simulink model "MVB1TestFlow"  (R2013b)
settings: Solver=ode45  StartTime=0.0  StopTime=6e-5  RelTol=1e-3
libraries: simulink x4
(part 1 of 2)
settings Model: Creator=qiji  LastModifiedBy=qiji
settings DataIOCC: SignalLoggingSaveFormat=ModelDataLogs
settings DebuggingCC: UnderspecifiedInitializationDetection=Simplified  MultiTaskDSMMsg=warning  MultiTaskCondExecSysMsg=none  SFUnusedDataAndEventsDiag=none
settings RTWCC: IncludeERTFirstTime=on
settings GRTTargetCC: CodeReplacementLibrary=None  CPPClassGenCompliant=on

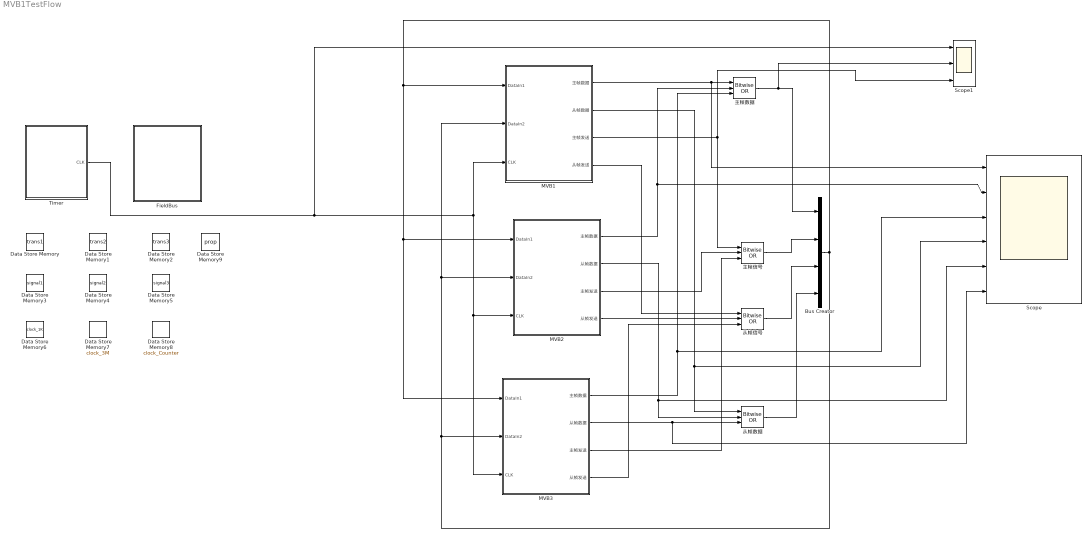
== system MVB1TestFlow ==
  Bus Creator : BusCreator
  Data Store Memory : DataStoreMemory  DataStoreName=trans1  ReadBeforeWriteMsg=warning  WriteAfterWriteMsg=warning  WriteAfterReadMsg=warning  OutDataTypeStr=boolean
  Data Store Memory1 : DataStoreMemory  DataStoreName=trans2  ReadBeforeWriteMsg=warning  WriteAfterWriteMsg=warning  WriteAfterReadMsg=warning  OutDataTypeStr=boolean
  Data Store Memory2 : DataStoreMemory  DataStoreName=trans3  ReadBeforeWriteMsg=warning  WriteAfterWriteMsg=warning  WriteAfterReadMsg=warning  OutDataTypeStr=boolean
  Data Store Memory3 : DataStoreMemory  DataStoreName=signal1  ReadBeforeWriteMsg=warning  WriteAfterWriteMsg=warning  WriteAfterReadMsg=warning  OutDataTypeStr=boolean
  Data Store Memory4 : DataStoreMemory  DataStoreName=signal2  ReadBeforeWriteMsg=warning  WriteAfterWriteMsg=warning  WriteAfterReadMsg=warning  OutDataTypeStr=boolean
  Data Store Memory5 : DataStoreMemory  DataStoreName=signal3  ReadBeforeWriteMsg=warning  WriteAfterWriteMsg=warning  WriteAfterReadMsg=warning  OutDataTypeStr=boolean
  Data Store Memory6 : DataStoreMemory  DataStoreName=clock_1K  ReadBeforeWriteMsg=warning  WriteAfterWriteMsg=warning  WriteAfterReadMsg=warning  OutDataTypeStr=boolean
  Data Store Memory7 : DataStoreMemory  DataStoreName=clock_3M  ReadBeforeWriteMsg=warning  WriteAfterWriteMsg=warning  WriteAfterReadMsg=warning  OutDataTypeStr=boolean
  Data Store Memory8 : DataStoreMemory  DataStoreName=clock_Counter  ReadBeforeWriteMsg=warning  WriteAfterWriteMsg=warning  WriteAfterReadMsg=warning  OutDataTypeStr=uint32
  Data Store Memory9 : DataStoreMemory  DataStoreName=prop  ReadBeforeWriteMsg=warning  WriteAfterWriteMsg=warning  WriteAfterReadMsg=warning  InitialValue=10  OutDataTypeStr=double
  FieldBus : Subsystem
  MVB1 : Subsystem
  MVB2 : Subsystem
  MVB3 : Subsystem
  Scope : Scope  NumInputPorts=6
      settings: YMin=0~0~0~0~0~0  YMax=3e+09~3e+09~3e+09~3e+09~3000000000~3e+09
  Scope1 : Scope  NumInputPorts=3
      settings: YMin=-5~-5~-5  YMax=5~5~5
  Timer : Subsystem
  主帧信号 : simulink/Logic and Bit Operations/Bitwise Operator  logicop=OR  UseBitMask=off  NumInputPorts=3  BitMask=bin2dec('11011001')  BitMaskRealWorld=Stored Integer
  主帧数据 : simulink/Logic and Bit Operations/Bitwise Operator  logicop=OR  UseBitMask=off  NumInputPorts=3  BitMask=bin2dec('11011001')  BitMaskRealWorld=Stored Integer
  从帧信号 : simulink/Logic and Bit Operations/Bitwise Operator  logicop=OR  UseBitMask=off  NumInputPorts=3  BitMask=bin2dec('11011001')  BitMaskRealWorld=Stored Integer
  从帧数据 : simulink/Logic and Bit Operations/Bitwise Operator  logicop=OR  UseBitMask=off  NumInputPorts=3  BitMask=bin2dec('11011001')  BitMaskRealWorld=Stored Integer
  wires:
  MVB1/1(主帧数据) -> Scope/1, 主帧数据/1
  MVB2/1(主帧数据) -> Scope/2, 主帧数据/2
  MVB3/1(主帧数据) -> Scope/3, 主帧数据/3
  MVB1/2(从帧数据) -> Scope/4, 从帧数据/1
  MVB2/2(从帧数据) -> Scope/5, 从帧数据/2
  MVB3/2(从帧数据) -> Scope/6, 从帧数据/3
  MVB1/3(主帧发送) -> 主帧信号/1, Scope1/3
  MVB2/3(主帧发送) -> 主帧信号/2
  MVB3/3(主帧发送) -> 主帧信号/3
  MVB1/4(从帧发送) -> 从帧信号/1
  MVB2/4(从帧发送) -> 从帧信号/2
  MVB3/4(从帧发送) -> 从帧信号/3
  主帧数据/1 -> Scope1/2, Bus Creator/1
  主帧信号/1 -> Bus Creator/2
  从帧信号/1 -> Bus Creator/3
  从帧数据/1 -> Bus Creator/4
  Bus Creator/1 -> MVB3/1(DataIn1), MVB2/1(DataIn1), MVB1/1(DataIn1), MVB3/2(DataIn2), MVB1/2(DataIn2), MVB2/2(DataIn2)
  Timer/1(CLK) -> Scope1/1, MVB1/3(CLK), MVB3/3(CLK), MVB2/3(CLK)

== system MVB1TestFlow/FieldBus ==
  FIELDBUS : Stateflow chart  TreatAsAtomicUnit=on

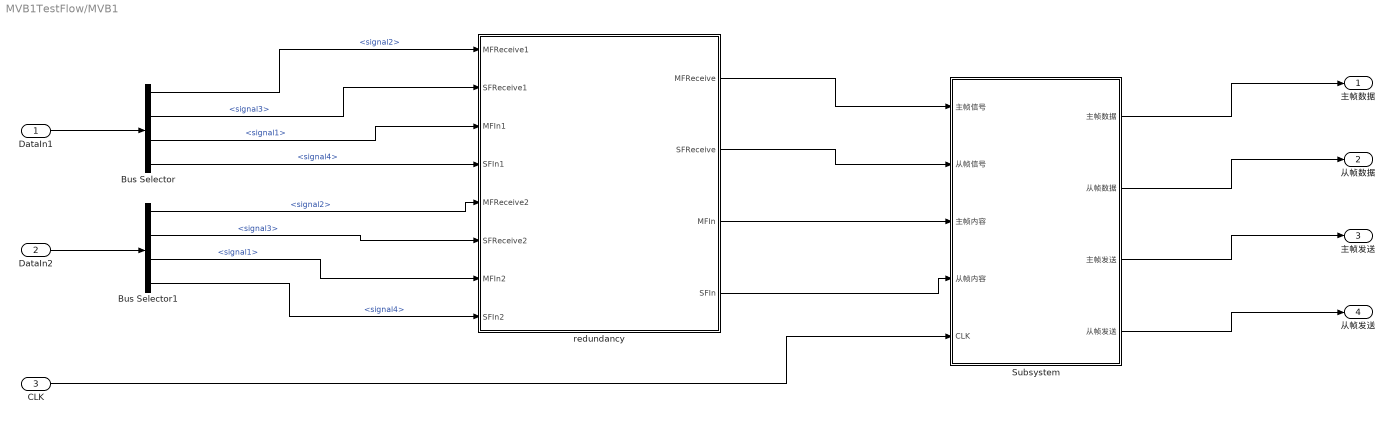
== system MVB1TestFlow/MVB1 ==
  DataIn1 : Inport  PortDimensions=4
  DataIn2 : Inport  Port=2  PortDimensions=4
  CLK : Inport  Port=3
  Bus Selector : BusSelector  OutputSignals=signal2,signal3,signal1,signal4
  Bus Selector1 : BusSelector  OutputSignals=signal2,signal3,signal1,signal4
  Subsystem : Subsystem
  redundancy : Stateflow chart  TreatAsAtomicUnit=on
  主帧数据 : Outport
  从帧数据 : Outport  Port=2
  主帧发送 : Outport  Port=3
  从帧发送 : Outport  Port=4
  wires:
  Subsystem/1(主帧数据) -> 主帧数据/1
  Subsystem/2(从帧数据) -> 从帧数据/1
  Subsystem/3(主帧发送) -> 主帧发送/1
  Subsystem/4(从帧发送) -> 从帧发送/1
  DataIn1/1 -> Bus Selector/1
  Bus Selector/3 -> redundancy/3(MFIn1)  "<signal1>"
  Bus Selector/1 -> redundancy/1(MFReceive1)  "<signal2>"
  Bus Selector/2 -> redundancy/2(SFReceive1)  "<signal3>"
  Bus Selector/4 -> redundancy/4(SFIn1)  "<signal4>"
  DataIn2/1 -> Bus Selector1/1
  redundancy/1(MFReceive) -> Subsystem/1(主帧信号)
  redundancy/2(SFReceive) -> Subsystem/2(从帧信号)
  redundancy/3(MFIn) -> Subsystem/3(主帧内容)
  redundancy/4(SFIn) -> Subsystem/4(从帧内容)
  Bus Selector1/1 -> redundancy/5(MFReceive2)  "<signal2>"
  Bus Selector1/2 -> redundancy/6(SFReceive2)  "<signal3>"
  Bus Selector1/3 -> redundancy/7(MFIn2)  "<signal1>"
  Bus Selector1/4 -> redundancy/8(SFIn2)  "<signal4>"
  CLK/1 -> Subsystem/5(CLK)

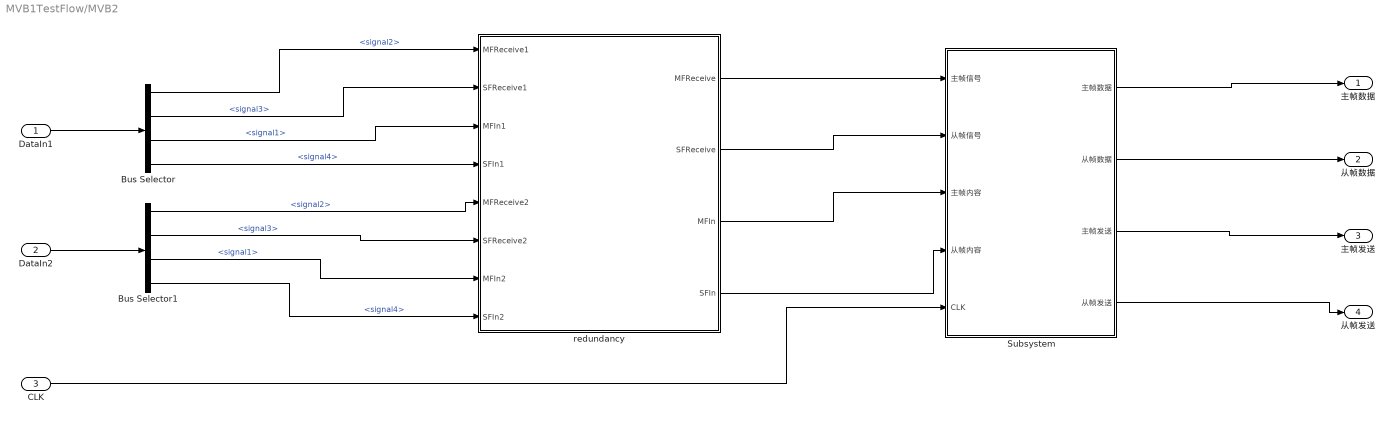
== system MVB1TestFlow/MVB2 ==
  DataIn1 : Inport  PortDimensions=4
  DataIn2 : Inport  Port=2  PortDimensions=4
  CLK : Inport  Port=3
  Bus Selector : BusSelector  OutputSignals=signal2,signal3,signal1,signal4
  Bus Selector1 : BusSelector  OutputSignals=signal2,signal3,signal1,signal4
  Subsystem : Subsystem
  redundancy : Stateflow chart  TreatAsAtomicUnit=on
  主帧数据 : Outport
  从帧数据 : Outport  Port=2
  主帧发送 : Outport  Port=3
  从帧发送 : Outport  Port=4
  wires:
  Subsystem/1(主帧数据) -> 主帧数据/1
  Subsystem/2(从帧数据) -> 从帧数据/1
  Subsystem/3(主帧发送) -> 主帧发送/1
  Subsystem/4(从帧发送) -> 从帧发送/1
  DataIn1/1 -> Bus Selector/1
  Bus Selector/3 -> redundancy/3(MFIn1)  "<signal1>"
  Bus Selector/1 -> redundancy/1(MFReceive1)  "<signal2>"
  Bus Selector/2 -> redundancy/2(SFReceive1)  "<signal3>"
  Bus Selector/4 -> redundancy/4(SFIn1)  "<signal4>"
  DataIn2/1 -> Bus Selector1/1
  redundancy/1(MFReceive) -> Subsystem/1(主帧信号)
  redundancy/2(SFReceive) -> Subsystem/2(从帧信号)
  redundancy/3(MFIn) -> Subsystem/3(主帧内容)
  redundancy/4(SFIn) -> Subsystem/4(从帧内容)
  Bus Selector1/1 -> redundancy/5(MFReceive2)  "<signal2>"
  Bus Selector1/2 -> redundancy/6(SFReceive2)  "<signal3>"
  Bus Selector1/3 -> redundancy/7(MFIn2)  "<signal1>"
  Bus Selector1/4 -> redundancy/8(SFIn2)  "<signal4>"
  CLK/1 -> Subsystem/5(CLK)

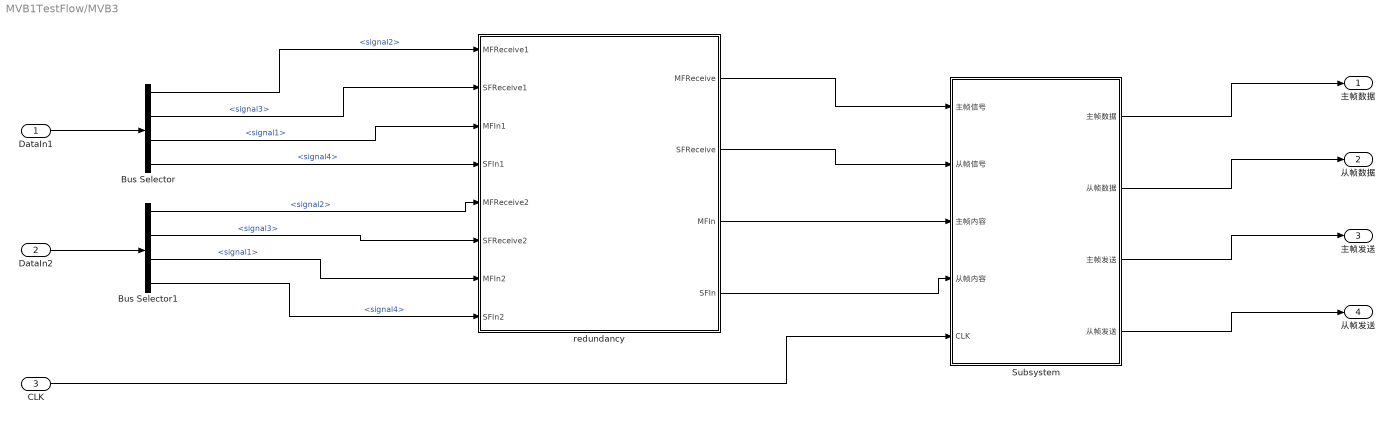
== system MVB1TestFlow/MVB3 ==
  DataIn1 : Inport  PortDimensions=4
  DataIn2 : Inport  Port=2  PortDimensions=4
  CLK : Inport  Port=3
  Bus Selector : BusSelector  OutputSignals=signal2,signal3,signal1,signal4
  Bus Selector1 : BusSelector  OutputSignals=signal2,signal3,signal1,signal4
  Subsystem : Subsystem
  redundancy : Stateflow chart  TreatAsAtomicUnit=on
  主帧数据 : Outport
  从帧数据 : Outport  Port=2
  主帧发送 : Outport  Port=3
  从帧发送 : Outport  Port=4
  wires:
  Subsystem/1(主帧数据) -> 主帧数据/1
  Subsystem/2(从帧数据) -> 从帧数据/1
  Subsystem/3(主帧发送) -> 主帧发送/1
  Subsystem/4(从帧发送) -> 从帧发送/1
  DataIn1/1 -> Bus Selector/1
  Bus Selector/3 -> redundancy/3(MFIn1)  "<signal1>"
  Bus Selector/1 -> redundancy/1(MFReceive1)  "<signal2>"
  Bus Selector/2 -> redundancy/2(SFReceive1)  "<signal3>"
  Bus Selector/4 -> redundancy/4(SFIn1)  "<signal4>"
  DataIn2/1 -> Bus Selector1/1
  redundancy/1(MFReceive) -> Subsystem/1(主帧信号)
  redundancy/2(SFReceive) -> Subsystem/2(从帧信号)
  redundancy/3(MFIn) -> Subsystem/3(主帧内容)
  redundancy/4(SFIn) -> Subsystem/4(从帧内容)
  Bus Selector1/1 -> redundancy/5(MFReceive2)  "<signal2>"
  Bus Selector1/2 -> redundancy/6(SFReceive2)  "<signal3>"
  Bus Selector1/3 -> redundancy/7(MFIn2)  "<signal1>"
  Bus Selector1/4 -> redundancy/8(SFIn2)  "<signal4>"
  CLK/1 -> Subsystem/5(CLK)

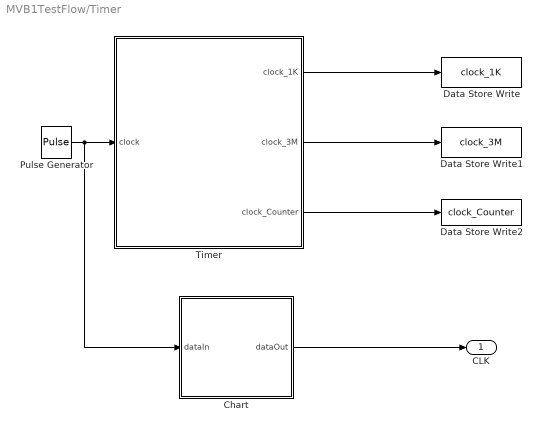
== system MVB1TestFlow/Timer ==
  Chart : Stateflow chart  TreatAsAtomicUnit=on
  Data Store Write : DataStoreWrite  DataStoreName=clock_1K
  Data Store Write1 : DataStoreWrite  DataStoreName=clock_3M
  Data Store Write2 : DataStoreWrite  DataStoreName=clock_Counter
  Pulse Generator : DiscretePulseGenerator  PulseType=Time based  Period=4.1666666667e-8  PulseWidth=50
  Timer : Stateflow chart  TreatAsAtomicUnit=on
  CLK : Outport  OutDataTypeStr=double
  wires:
  Timer/3(clock_Counter) -> Data Store Write2/1
  Timer/2(clock_3M) -> Data Store Write1/1
  Timer/1(clock_1K) -> Data Store Write/1
  Pulse Generator/1 -> Chart/1(dataIn), Timer/1(clock)
  Chart/1(dataOut) -> CLK/1

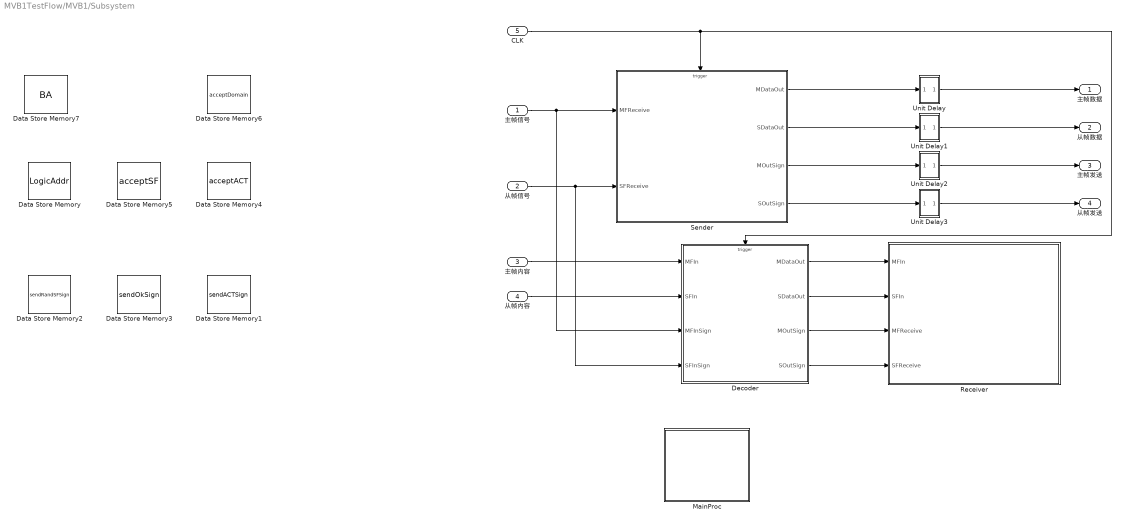
== system MVB1TestFlow/MVB1/Subsystem ==
  主帧信号 : Inport
  从帧信号 : Inport  Port=2
  主帧内容 : Inport  Port=3
  从帧内容 : Inport  Port=4
  CLK : Inport  Port=5
  Data Store Memory : DataStoreMemory  DataStoreName=LogicAddr  ReadBeforeWriteMsg=warning  WriteAfterWriteMsg=warning  WriteAfterReadMsg=warning  InitialValue=1  OutDataTypeStr=uint32
  Data Store Memory1 : DataStoreMemory  DataStoreName=sendACTSign  ReadBeforeWriteMsg=warning  WriteAfterWriteMsg=warning  WriteAfterReadMsg=warning  OutDataTypeStr=boolean
  Data Store Memory2 : DataStoreMemory  DataStoreName=sendRandSFSign  ReadBeforeWriteMsg=warning  WriteAfterWriteMsg=warning  WriteAfterReadMsg=warning  OutDataTypeStr=boolean
  Data Store Memory3 : DataStoreMemory  DataStoreName=sendOkSign  ReadBeforeWriteMsg=warning  WriteAfterWriteMsg=warning  WriteAfterReadMsg=warning  OutDataTypeStr=boolean
  Data Store Memory4 : DataStoreMemory  DataStoreName=acceptACT  ReadBeforeWriteMsg=warning  WriteAfterWriteMsg=warning  WriteAfterReadMsg=warning  InitialValue=false  OutDataTypeStr=boolean
  Data Store Memory5 : DataStoreMemory  DataStoreName=acceptSF  ReadBeforeWriteMsg=warning  WriteAfterWriteMsg=warning  WriteAfterReadMsg=warning  InitialValue=false  OutDataTypeStr=boolean
  Data Store Memory6 : DataStoreMemory  DataStoreName=acceptDomain  ReadBeforeWriteMsg=warning  WriteAfterWriteMsg=warning  WriteAfterReadMsg=warning  InitialValue=false  OutDataTypeStr=boolean
  Data Store Memory7 : DataStoreMemory  DataStoreName=BA  ReadBeforeWriteMsg=warning  WriteAfterWriteMsg=warning  WriteAfterReadMsg=warning  InitialValue=true  OutDataTypeStr=boolean
  Decoder : Stateflow chart  TreatAsAtomicUnit=on
  MainProc : Stateflow chart  TreatAsAtomicUnit=on
  Receiver : Stateflow chart  TreatAsAtomicUnit=on
  Sender : Stateflow chart  TreatAsAtomicUnit=on
  Unit Delay : Subsystem
  Unit Delay1 : Subsystem
  Unit Delay2 : Subsystem
  Unit Delay3 : Subsystem
  主帧数据 : Outport
  从帧数据 : Outport  Port=2
  主帧发送 : Outport  Port=3
  从帧发送 : Outport  Port=4
  wires:
  主帧信号/1 -> Decoder/3(MFInSign), Sender/1(MFReceive)
  Sender/3(MOutSign) -> Unit Delay2/1(In1)
  Sender/2(SDataOut) -> Unit Delay1/1(In1)
  Unit Delay3/1(Out) -> 从帧发送/1
  从帧信号/1 -> Decoder/4(SFInSign), Sender/2(SFReceive)
  Unit Delay1/1(Out) -> 从帧数据/1
  Sender/4(SOutSign) -> Unit Delay3/1(In1)
  从帧内容/1 -> Decoder/2(SFIn)
  Sender/1(MDataOut) -> Unit Delay/1(In1)
  Unit Delay2/1(Out) -> 主帧发送/1
  主帧内容/1 -> Decoder/1(MFIn)
  CLK/1 -> Decoder/Trigger, Sender/Trigger
  Decoder/1(MDataOut) -> Receiver/1(MFIn)
  Decoder/2(SDataOut) -> Receiver/2(SFIn)
  Decoder/3(MOutSign) -> Receiver/3(MFReceive)
  Decoder/4(SOutSign) -> Receiver/4(SFReceive)
  Unit Delay/1(Out) -> 主帧数据/1

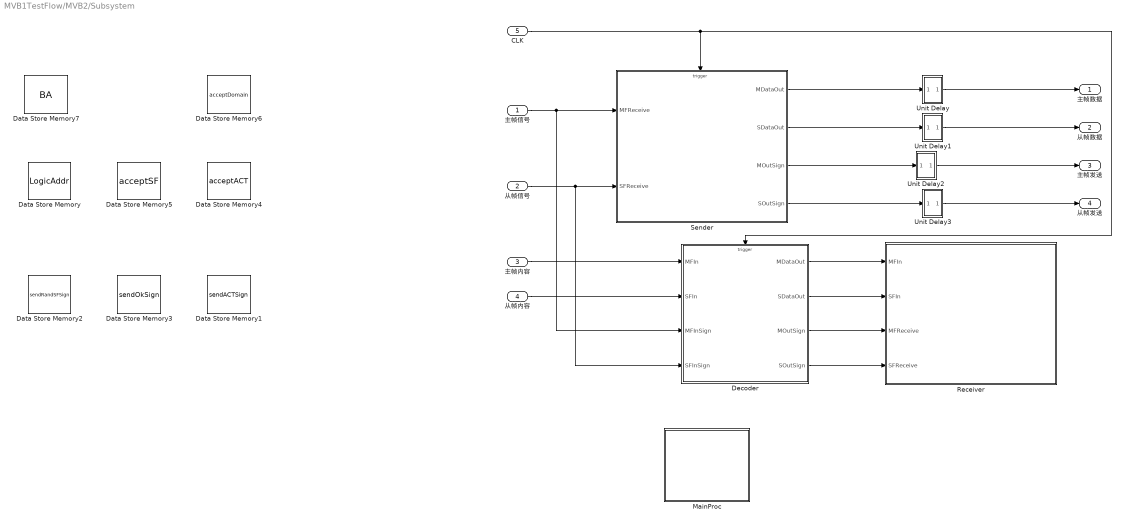
== system MVB1TestFlow/MVB2/Subsystem ==
  主帧信号 : Inport
  从帧信号 : Inport  Port=2
  主帧内容 : Inport  Port=3
  从帧内容 : Inport  Port=4
  CLK : Inport  Port=5
  Data Store Memory : DataStoreMemory  DataStoreName=LogicAddr  ReadBeforeWriteMsg=warning  WriteAfterWriteMsg=warning  WriteAfterReadMsg=warning  InitialValue=2  OutDataTypeStr=uint32
  Data Store Memory1 : DataStoreMemory  DataStoreName=sendACTSign  ReadBeforeWriteMsg=warning  WriteAfterWriteMsg=warning  WriteAfterReadMsg=warning  OutDataTypeStr=boolean
  Data Store Memory2 : DataStoreMemory  DataStoreName=sendRandSFSign  ReadBeforeWriteMsg=warning  WriteAfterWriteMsg=warning  WriteAfterReadMsg=warning  OutDataTypeStr=boolean
  Data Store Memory3 : DataStoreMemory  DataStoreName=sendOkSign  ReadBeforeWriteMsg=warning  WriteAfterWriteMsg=warning  WriteAfterReadMsg=warning  OutDataTypeStr=boolean
  Data Store Memory4 : DataStoreMemory  DataStoreName=acceptACT  ReadBeforeWriteMsg=warning  WriteAfterWriteMsg=warning  WriteAfterReadMsg=warning  InitialValue=false  OutDataTypeStr=boolean
  Data Store Memory5 : DataStoreMemory  DataStoreName=acceptSF  ReadBeforeWriteMsg=warning  WriteAfterWriteMsg=warning  WriteAfterReadMsg=warning  InitialValue=false  OutDataTypeStr=boolean
  Data Store Memory6 : DataStoreMemory  DataStoreName=acceptDomain  ReadBeforeWriteMsg=warning  WriteAfterWriteMsg=warning  WriteAfterReadMsg=warning  InitialValue=false  OutDataTypeStr=boolean
  Data Store Memory7 : DataStoreMemory  DataStoreName=BA  ReadBeforeWriteMsg=warning  WriteAfterWriteMsg=warning  WriteAfterReadMsg=warning  InitialValue=true  OutDataTypeStr=boolean
  Decoder : Stateflow chart  TreatAsAtomicUnit=on
  MainProc : Stateflow chart  TreatAsAtomicUnit=on
  Receiver : Stateflow chart  TreatAsAtomicUnit=on
  Sender : Stateflow chart  TreatAsAtomicUnit=on
  Unit Delay : Subsystem
  Unit Delay1 : Subsystem
  Unit Delay2 : Subsystem
  Unit Delay3 : Subsystem
  主帧数据 : Outport
  从帧数据 : Outport  Port=2
  主帧发送 : Outport  Port=3
  从帧发送 : Outport  Port=4
  wires:
  主帧信号/1 -> Decoder/3(MFInSign), Sender/1(MFReceive)
  Sender/3(MOutSign) -> Unit Delay2/1(In1)
  Sender/2(SDataOut) -> Unit Delay1/1(In1)
  Unit Delay3/1(Out) -> 从帧发送/1
  从帧信号/1 -> Decoder/4(SFInSign), Sender/2(SFReceive)
  Unit Delay1/1(Out) -> 从帧数据/1
  Sender/4(SOutSign) -> Unit Delay3/1(In1)
  从帧内容/1 -> Decoder/2(SFIn)
  Sender/1(MDataOut) -> Unit Delay/1(In1)
  Unit Delay/1(Out) -> 主帧数据/1
  Unit Delay2/1(Out) -> 主帧发送/1
  主帧内容/1 -> Decoder/1(MFIn)
  CLK/1 -> Decoder/Trigger, Sender/Trigger
  Decoder/1(MDataOut) -> Receiver/1(MFIn)
  Decoder/2(SDataOut) -> Receiver/2(SFIn)
  Decoder/3(MOutSign) -> Receiver/3(MFReceive)
  Decoder/4(SOutSign) -> Receiver/4(SFReceive)

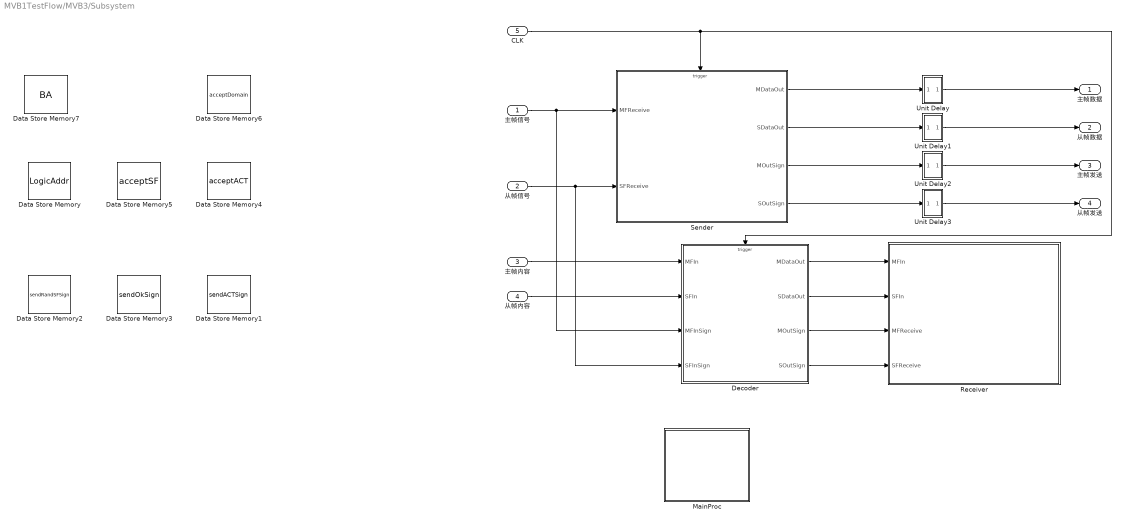
== system MVB1TestFlow/MVB3/Subsystem ==
  主帧信号 : Inport
  从帧信号 : Inport  Port=2
  主帧内容 : Inport  Port=3
  从帧内容 : Inport  Port=4
  CLK : Inport  Port=5
  Data Store Memory : DataStoreMemory  DataStoreName=LogicAddr  ReadBeforeWriteMsg=warning  WriteAfterWriteMsg=warning  WriteAfterReadMsg=warning  InitialValue=3  OutDataTypeStr=uint32
  Data Store Memory1 : DataStoreMemory  DataStoreName=sendACTSign  ReadBeforeWriteMsg=warning  WriteAfterWriteMsg=warning  WriteAfterReadMsg=warning  OutDataTypeStr=boolean
  Data Store Memory2 : DataStoreMemory  DataStoreName=sendRandSFSign  ReadBeforeWriteMsg=warning  WriteAfterWriteMsg=warning  WriteAfterReadMsg=warning  OutDataTypeStr=boolean
  Data Store Memory3 : DataStoreMemory  DataStoreName=sendOkSign  ReadBeforeWriteMsg=warning  WriteAfterWriteMsg=warning  WriteAfterReadMsg=warning  OutDataTypeStr=boolean
  Data Store Memory4 : DataStoreMemory  DataStoreName=acceptACT  ReadBeforeWriteMsg=warning  WriteAfterWriteMsg=warning  WriteAfterReadMsg=warning  InitialValue=false  OutDataTypeStr=boolean
  Data Store Memory5 : DataStoreMemory  DataStoreName=acceptSF  ReadBeforeWriteMsg=warning  WriteAfterWriteMsg=warning  WriteAfterReadMsg=warning  InitialValue=false  OutDataTypeStr=boolean
  Data Store Memory6 : DataStoreMemory  DataStoreName=acceptDomain  ReadBeforeWriteMsg=warning  WriteAfterWriteMsg=warning  WriteAfterReadMsg=warning  InitialValue=false  OutDataTypeStr=boolean
  Data Store Memory7 : DataStoreMemory  DataStoreName=BA  ReadBeforeWriteMsg=warning  WriteAfterWriteMsg=warning  WriteAfterReadMsg=warning  InitialValue=true  OutDataTypeStr=boolean
  Decoder : Stateflow chart  TreatAsAtomicUnit=on
  MainProc : Stateflow chart  TreatAsAtomicUnit=on
  Receiver : Stateflow chart  TreatAsAtomicUnit=on
  Sender : Stateflow chart  TreatAsAtomicUnit=on
  Unit Delay : Subsystem
  Unit Delay1 : Subsystem
  Unit Delay2 : Subsystem
  Unit Delay3 : Subsystem
  主帧数据 : Outport
  从帧数据 : Outport  Port=2
  主帧发送 : Outport  Port=3
  从帧发送 : Outport  Port=4
  wires:
  主帧信号/1 -> Decoder/3(MFInSign), Sender/1(MFReceive)
  Sender/3(MOutSign) -> Unit Delay2/1(In1)
  Sender/2(SDataOut) -> Unit Delay1/1(In1)
  Unit Delay3/1(Out) -> 从帧发送/1
  从帧信号/1 -> Decoder/4(SFInSign), Sender/2(SFReceive)
  Unit Delay1/1(Out) -> 从帧数据/1
  Sender/4(SOutSign) -> Unit Delay3/1(In1)
  从帧内容/1 -> Decoder/2(SFIn)
  Sender/1(MDataOut) -> Unit Delay/1(In1)
  Unit Delay/1(Out) -> 主帧数据/1
  Unit Delay2/1(Out) -> 主帧发送/1
  主帧内容/1 -> Decoder/1(MFIn)
  CLK/1 -> Decoder/Trigger, Sender/Trigger
  Decoder/1(MDataOut) -> Receiver/1(MFIn)
  Decoder/2(SDataOut) -> Receiver/2(SFIn)
  Decoder/3(MOutSign) -> Receiver/3(MFReceive)
  Decoder/4(SOutSign) -> Receiver/4(SFReceive)

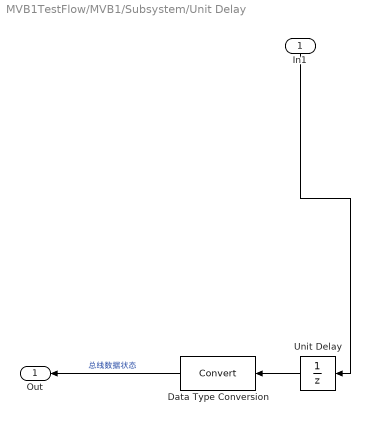
== system MVB1TestFlow/MVB1/Subsystem/Unit Delay ==
  In1 : Inport
  Data Type Conversion : DataTypeConversion
  Unit Delay : UnitDelay  SampleTime=-1
  Out : Outport
  wires:
  Data Type Conversion/1 -> Out/1  "总线数据状态"
  Unit Delay/1 -> Data Type Conversion/1
  In1/1 -> Unit Delay/1

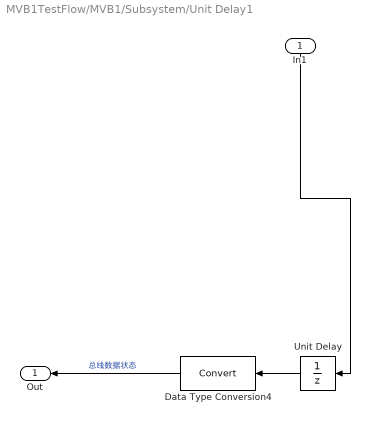
== system MVB1TestFlow/MVB1/Subsystem/Unit Delay1 ==
  In1 : Inport
  Data Type Conversion4 : DataTypeConversion
  Unit Delay : UnitDelay  SampleTime=-1
  Out : Outport
  wires:
  In1/1 -> Unit Delay/1
  Unit Delay/1 -> Data Type Conversion4/1
  Data Type Conversion4/1 -> Out/1  "总线数据状态"

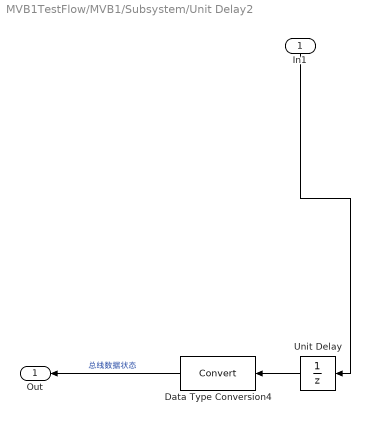
== system MVB1TestFlow/MVB1/Subsystem/Unit Delay2 ==
  In1 : Inport
  Data Type Conversion4 : DataTypeConversion
  Unit Delay : UnitDelay  SampleTime=-1
  Out : Outport
  wires:
  Data Type Conversion4/1 -> Out/1  "总线数据状态"
  Unit Delay/1 -> Data Type Conversion4/1
  In1/1 -> Unit Delay/1

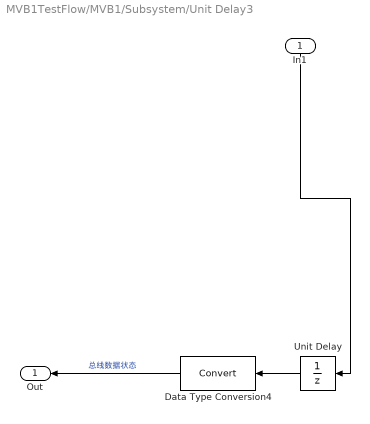
== system MVB1TestFlow/MVB1/Subsystem/Unit Delay3 ==
  In1 : Inport
  Data Type Conversion4 : DataTypeConversion
  Unit Delay : UnitDelay  SampleTime=-1
  Out : Outport
  wires:
  Data Type Conversion4/1 -> Out/1  "总线数据状态"
  Unit Delay/1 -> Data Type Conversion4/1
  In1/1 -> Unit Delay/1

== system MVB1TestFlow/MVB2/Subsystem/Unit Delay ==
  In1 : Inport
  Data Type Conversion : DataTypeConversion
  Unit Delay : UnitDelay  SampleTime=-1
  Out : Outport
  wires:
  Data Type Conversion/1 -> Out/1  "总线数据状态"
  Unit Delay/1 -> Data Type Conversion/1
  In1/1 -> Unit Delay/1

== system MVB1TestFlow/MVB2/Subsystem/Unit Delay1 ==
  In1 : Inport
  Data Type Conversion : DataTypeConversion
  Unit Delay : UnitDelay  SampleTime=-1
  Out : Outport
  wires:
  Data Type Conversion/1 -> Out/1  "总线数据状态"
  Unit Delay/1 -> Data Type Conversion/1
  In1/1 -> Unit Delay/1

== system MVB1TestFlow/MVB2/Subsystem/Unit Delay2 ==
  In1 : Inport
  Data Type Conversion : DataTypeConversion
  Unit Delay : UnitDelay  SampleTime=-1
  Out : Outport
  wires:
  Data Type Conversion/1 -> Out/1  "总线数据状态"
  Unit Delay/1 -> Data Type Conversion/1
  In1/1 -> Unit Delay/1

== system MVB1TestFlow/MVB2/Subsystem/Unit Delay3 ==
  In1 : Inport
  Data Type Conversion : DataTypeConversion
  Unit Delay : UnitDelay  SampleTime=-1
  Out : Outport
  wires:
  Data Type Conversion/1 -> Out/1  "总线数据状态"
  Unit Delay/1 -> Data Type Conversion/1
  In1/1 -> Unit Delay/1

== system MVB1TestFlow/MVB3/Subsystem/Unit Delay ==
  In1 : Inport
  Data Type Conversion : DataTypeConversion
  Unit Delay : UnitDelay  SampleTime=-1
  Out : Outport
  wires:
  Data Type Conversion/1 -> Out/1  "总线数据状态"
  Unit Delay/1 -> Data Type Conversion/1
  In1/1 -> Unit Delay/1

== system MVB1TestFlow/MVB3/Subsystem/Unit Delay1 ==
  In1 : Inport
  Data Type Conversion : DataTypeConversion
  Unit Delay : UnitDelay  SampleTime=-1
  Out : Outport
  wires:
  Data Type Conversion/1 -> Out/1  "总线数据状态"
  Unit Delay/1 -> Data Type Conversion/1
  In1/1 -> Unit Delay/1

== system MVB1TestFlow/MVB3/Subsystem/Unit Delay2 ==
  In1 : Inport
  Data Type Conversion : DataTypeConversion
  Unit Delay : UnitDelay  SampleTime=-1
  Out : Outport
  wires:
  Data Type Conversion/1 -> Out/1  "总线数据状态"
  Unit Delay/1 -> Data Type Conversion/1
  In1/1 -> Unit Delay/1

== system MVB1TestFlow/MVB3/Subsystem/Unit Delay3 ==
  In1 : Inport
  Data Type Conversion : DataTypeConversion
  Unit Delay : UnitDelay  SampleTime=-1
  Out : Outport
  wires:
  Data Type Conversion/1 -> Out/1  "总线数据状态"
  Unit Delay/1 -> Data Type Conversion/1
  In1/1 -> Unit Delay/1

== stateflow chart MVB1TestFlow/FieldBus/FIELDBUS ==
  state IDLE
  state busy
  state space
  state turnFalse [function]
    (default) -> (junction 45) : {
        | trans1 = false;
        | trans2 = false;
        | trans3 = false;
        | }
  state r = pull(a, b, c) [function]
    (default) -> (junction 17)
    (junction 17) -> (junction 19) [order 1] : [a==true]{trans1=true; r=1;}
    (junction 17) -> (junction 21) [order 2]
    (junction 21) -> (junction 22) [order 1] : [b==true]{trans2=true; r=1;}
    (junction 21) -> (junction 24) [order 2]
    (junction 24) -> (junction 23) : [c==true]{trans3=true;r=1}
  state init [function]
    (default) -> (junction 40) : {
        | trans1 = false;
        | trans2 = false;
        | trans3 = false;
        | }
  IDLE -> busy : [pull(signal1, signal2, signal3)]
  (default) -> IDLE
  busy -> space : {t = clock_Counter}
  space -> IDLE : [clock_Counter - t > (50/prop)]{turnFalse()}
  data: r function_output double; a function_input double; b function_input double; c function_input double; t local uint32; clock_Counter data_store_memory; trans1 data_store_memory; trans2 data_store_memory; trans3 data_store_memory; signal1 data_store_memory; signal2 data_store_memory; signal3 data_store_memory; prop data_store_memory

== stateflow chart MVB1TestFlow/Timer/Timer ==
  state ClockManager
    note: 时钟模块
    state initTimer [function]
      (default) -> (junction 13) : {
          | clock1K_Counter = uint32(0);
          | clock3M_Counter = uint32(0);
          | clock_Counter = uint32(0);
          | clock_1K = true;
          | clock_3M = true;
          | }
    state ClockStart
    state Devider
      state startDevider
      startDevider -> (junction 7) : [clock==1]
      (junction 7) -> (junction 8) [order 1] : [clock1K_Counter == 24000]
          | {
          | clock_1K = ~clock_1K;
          | clock1K_Counter = uint32(0);
          | }
      (junction 7) -> (junction 10) [order 2]
      (junction 8) -> (junction 10)
      (default) -> startDevider
      (junction 10) -> (junction 11) [order 1] : [clock3M_Counter == (500/prop)]
          | {
          | clock_3M = 1 - clock_3M;
          | clock3M_Counter = uint32(0);
          | }
      (junction 10) -> (junction 15) [order 2]
      (junction 15) -> startDevider : {
          | clock3M_Counter = clock3M_Counter + 1;
          | clock1K_Counter = clock1K_Counter + 1;
          | clock_Counter = clock_Counter + 1;
          | }
      (junction 11) -> (junction 15)
    (default) -> ClockStart
    ClockStart -> Devider : {
        | initTimer()
        | }
  data: clock1K_Counter local uint32; clock3M_Counter local uint32; clock_1K output boolean; clock_3M output boolean; clock_Counter output uint32; clock input double; prop data_store_memory

== stateflow chart MVB1TestFlow/MVB1/Subsystem/Sender ==
  state init [function]
    note: 请求随机从帧
        | 请求随机从帧
        | 请求2号的信息
        | 请求转移到2号
    note: SFT(1)代表随机的从帧
        | SFT(2)代表回复接受主权
        | SFT(3)代表回复设备LAT和BA
    (default) -> (junction 100) : {
        | BA = true;
        | MFIndex = 1;
        | isMaster = true;
        | SendSignal = false;
        | MFT(1) = getMF(0, 3);
        | MFT(2) = getMF(0, 2);
        | MFT(3) = getMF(15, 2);
        | MFT(4) = getMF(8, 2);
        | MFT(5) = 1;
        | SFT(1) = getSF(777);
        | SFT(2) = getSF(32768);
        | SFT(3) = getSF(16512);
        | clock_3M_shang = false;
        | sendRandSFSign = false;
        | sendACTSign = false;
        | sendRandSFSign = false;
        | }
  state SFSender [parallel]
    settings: executionOrder=1
    note: send**Signd的置位在接收到了请求数据的主帧后置位
    state sender [parallel]
      settings: executionOrder=1
      state wait
      state sendInfo
      state sendRandomSF
      state sendOK
      state transmission
        entry:
        SOutSign = true;
      (default) -> SFSender.sender.wait
      SFSender.sender.wait -> sendRandomSF [order 1] : [sendRandSFSign == true]
      SFSender.sender.wait -> sendOK [order 2] : [sendOkSign == true]
          | {
          | isMaster = true;
          | }
      SFSender.sender.wait -> sendInfo [order 3] : [sendACTSign == true]
      sendInfo -> SFSender.sender.transmission : {SFIndex = 3;
          | sendACTSign = false;}
      sendRandomSF -> SFSender.sender.transmission : {SFIndex = 1;
          | sendRandSFSign = false;}
      sendOK -> SFSender.sender.transmission : {SFIndex = 2;
          | sendOkSign = false;
          | init();
          | BA = true;
          | }
      SFSender.sender.transmission -> SFSender.sender : exit(SendHolder.hold)
          | {SDataOut = uint32(0);
          | SOutSign = false;
          | }
    state SendHolder [parallel]
      settings: executionOrder=2
      state hold
        entry:
        count = 0;
        hold -> hold [order 1] : CLK
            | {
            | SDataOut = bitoperate.getbit(input);
            | input = bitoperate.shiftbit(input, uint32(1));
            | count = count + 1;
            | }
      state end
      (default) -> end
      hold -> end [order 1] : [count == 32]
      end -> hold : enter(sender.transmission)
          | {
          | input =  ManchesterEncoding(SFT(SFIndex));
          | count = 0;
          | }
  state MFSender [parallel]
    settings: executionOrder=2
    state sender [parallel]
      settings: executionOrder=1
      state sleep
      state wait
        entry:
        signal1 = true
      state transmission
        entry:
        signal1 = false;
        [acceptSF, acceptACT, acceptDomain] = setAcceptSignal(MFT(MFIndex));
      (default) -> sleep : {
          | init();
          | }
      sleep -> MFSender.sender.wait : [BA==true && clock_3M ~= clock_3M_shang]
          | {
          | clock_3M_shang = clock_3M;
          | }
      MFSender.sender.transmission -> sleep : exit(buffer.full)
          | {
          | MFIndex = MFIndex + 1;
          | }
      MFSender.sender.wait -> MFSender.sender.transmission : [trans1 == true]
    state buffer [parallel]
      settings: executionOrder=2
      state full
        entry:
        count = 0;
        full -> full [order 1] : CLK
            | {
            | MDataOut = bitoperate.getbit(input);
            | input = bitoperate.shiftbit(input, uint32(1));
            | count = count + 1;
            | }
      state empty
      (default) -> empty
      full -> empty [order 1] : [count == 32]
          | {
          | MDataOut = uint32(0);
          | MOutSign = false;
          | }
      empty -> full : enter(sender.transmission)
          | {
          | input =  ManchesterEncoding(MFT(MFIndex));
          | count = 0;
          | MOutSign = true;
          | }
  state bitoperate [group]
  (default) -> MFSender
  data: f_code function_input; addr function_input; r function_output; addr function_input; r function_output; input local uint32; count local double; SFIndex local double; dataIn function_input uint32; SF function_output boolean; ACT function_output; Domain function_output; input local uint32; count local double; data function_input uint32; r function_output uint32; r function_output uint32; data function_input uint32; num function_input uint32; r function_output uint32; data function_input uint32; num function_input uint32; r function_output uint32; MFReceive input boolean; MDataOut output uint32; clock_3M data_store_memory; clock_Counter data_store_memory; MFIndex local; MFT local uint32 size=5; trans1 data_store_memory; signal1 data_store_memory; SFReceive input boolean; sendOkSign data_store_memory; sendRandSFSign data_store_memory; sendACTSign data_store_memory; SFT local uint32 size=3; SDataOut output uint32; MOutSign output boolean; SOutSign output boolean; isMaster local boolean; acceptSF data_store_memory; BA data_store_memory; clock_3M_shang local boolean; acceptACT data_store_memory; acceptDomain data_store_memory; prop data_store_memory
  events: CLK input EITHER_EDGE_EVENT
  function r = getMF(f_code, addr):
    | function r = getMF(f_code, addr)
    | r = 3340042240;
    | r = r + bitshift(uint32(f_code), 12);
    | r = r + addr;
  function r = getSF(addr):
    | function r = getSF(addr)
    | r = 2833448960;
    | r = r + addr;
  function judgeMaster:
    | function judgeMaster
    | % 如果
    | if isMaster == true && SFIndex == 2
    |     isMaster = false;
    | end
  function [SF, ACT, Domain] = setAcceptSignal(dataIn):
    | function [SF, ACT, Domain] = setAcceptSignal(dataIn)
    | % 右移12位 仅保留帧头和fcode
    | dataInExAddr = bitshift(uint32(dataIn), -12);
    | % 先右移16位再左移4位 仅仅保留帧头
    | dataInStart = bitshift(bitshift(uint32(dataIn), -16), 4);
    | % 相减得到fcode
    | fcode = double(dataInExAddr - dataInStart);
    | SF = false;
    | Domain = false;
    | ACT = false;
    | if fcode == 0
    |     SF = true;
    | elseif fcode == 15
    |     ACT = true;
    | else
    |     Domain = true;
    | end
  function r = ManchesterEncoding(data):
    | function r = ManchesterEncoding(data)
    | r = data;
    | for i = 1:16
    |     x = bitget(data, i);
    |     if x == 0
    |         r = bitset(r, i*2-1, 1);
    |         r = bitset(r, i*2, 0);
    |     else
    |         r = bitset(r, i*2-1, 0);
    |         r = bitset(r, i*2, 1);
    |     end
    | end
  function r = ManchesterDecoding(data):
    | function r = ManchesterDecoding(data)
    | r = uint32(0);
    | for i = (1:2:32)
    |     x0 = bitget(data, i);
    |     x1 = bitget(data, i+1);
    |     if x0==0 && x1==1
    |         r = bitset(r, (i+1)/2, 1);
    |     else
    |         r = bitset(r, (i+1)/2, 0);
    |     end
    | end
  function r = getbit(num):
    | function r = getbit(num)
    | r = bitget(num, 32);
  function r = shiftbit(data, num):
    | function r = shiftbit(data, num)
    | r = bitshift(data, num);
    | %for i=1:cnt
    | %   r = bitset(r, i, 0);
    | %end

== stateflow chart MVB1TestFlow/MVB1/Subsystem/MainProc ==
  note: 上一个主帧接收后1.3ms没有收到主帧产生一个主帧超时的通知。
  state Timer [parallel]
    settings: executionOrder=1
    state Timer
      entry:
      t = clock_Counter;
      timeOut = false;
    state start
    state TimeOut
      entry:
      timeOut = true;
    start -> Timer.Timer : [startTimer == true]
    (default) -> start
    Timer.Timer -> start [order 1] : [endTimer == true]
    Timer.TimeOut -> start
    Timer.Timer -> Timer.TimeOut [order 2] : [clock_Counter - t > (1300/prop)]
  state mainproc [parallel]
    settings: executionOrder=2
    state StandbyEquip
      entry:
      startTimer = true;
      endTimer = false;
    state MainEquip
    state TimeOut
    state wait4ACT
    note: 等待其他设备返回ACT
    note: 等待其他设备返回OK，receiver在接收到OK以后立马放弃主权
    state TempEquip
      entry:
      startTimer = true;
      endTimer = false;
    (default) -> StandbyEquip
    mainproc.TimeOut -> StandbyEquip
    StandbyEquip -> mainproc.TimeOut [order 2] : [timeOut == true]
    TempEquip -> StandbyEquip [order 1] : [BA == false]
        | {
        | endTimer = true;
        | startTimer = false;
        | }
    StandbyEquip -> MainEquip [order 1] : [BA == true && ACT == true]
        | {
        | endTimer = true;
        | startTimer = false;
        | }
    MainEquip -> wait4ACT : [acceptACT == true]
        | {
        | t = clock_Counter;
        | }
    TempEquip -> mainproc.TimeOut [order 2] : [timeOut == true]
    wait4ACT -> TempEquip : [acceptDomain == true]
        | {
        | t = clock_Counter;
        | }
  data: BA data_store_memory; ACT local boolean =true; acceptACT data_store_memory; acceptDomain data_store_memory; t local uint32; clock_Counter data_store_memory; startTimer local boolean; timeOut local boolean; endTimer local boolean; prop data_store_memory

== stateflow chart MVB1TestFlow/MVB2/Subsystem/Decoder ==
  state decodeSF
    decodeSF -> decodeSF [order 1] : CLK
        | {
        | ans = bitoperate.shiftbit(ans, 1) + SFIn;
        | count++;
        | }
  state bitoperate [group]
  state start
  state decodeMF
    decodeMF -> decodeMF [order 1] : CLK
        | {
        | ans = bitoperate.shiftbit(ans, 1) + MFIn;
        | count++;
        | }
  start -> decodeSF [order 2] : [SFInSign == true]
      | {
      | ans = 0;
      | count = 0;
      | SDataOut = 0;
      | SOutSign = true;
      | ans = bitoperate.shiftbit(ans, 1) + SFIn;
      | count++;
      | }
  decodeSF -> start [order 1] : [count==32]
      | {
      | ans = ManchesterDecoding(ans);
      | SDataOut = ans;
      | SOutSign = false;
      | }
  start -> decodeMF [order 1] : [MFInSign==true]
      | {
      | ans = 0;
      | count = 0;
      | MDataOut = 0;
      | MOutSign = true
      | ans = bitoperate.shiftbit(ans, 1) + MFIn;
      | count++;
      | }
  (default) -> start
  decodeMF -> start [order 1] : [count==32]
      | {
      | ans = ManchesterDecoding(ans);
      | MDataOut = ans;
      | MOutSign = false;
      | }
  data: num function_input uint32; r function_output uint32; data function_input uint32; num function_input uint32; r function_output uint32; r function_output uint32; data function_input uint32; MFIn input uint32; SFIn input uint32; MDataOut output uint32; MFInSign input boolean; count local uint32; SFInSign input boolean; SDataOut output uint32; MOutSign output boolean; SOutSign output boolean; ans local uint32
  events: CLK input EITHER_EDGE_EVENT
  function r = getbit(num):
    | function r = getbit(num)
    | r = bitget(num, 32);
  function r = shiftbit(data, num):
    | function r = shiftbit(data, num)
    | r = bitshift(data, num);
    | %for i=1:cnt
    | %   r = bitset(r, i, 0);
    | %end
  function r = ManchesterDecoding(data):
    | function r = ManchesterDecoding(data)
    | r = uint32(0);
    | for i = (1:2:32)
    |     x0 = bitget(data, i);
    |     x1 = bitget(data, i+1);
    |     if x0==0 && x1==1
    |         r = bitset(r, (i+1)/2, 1);
    |     else
    |         r = bitset(r, (i+1)/2, 0);
    |     end
    | end

== stateflow chart MVB1TestFlow/MVB2/Subsystem/MainProc ==
  note: 上一个主帧接收后1.3ms没有收到主帧产生一个主帧超时的通知。
  state Timer [parallel]
    settings: executionOrder=1
    state Timer
      entry:
      t = clock_Counter;
      timeOut = false;
    state start
    state TimeOut
      entry:
      timeOut = true;
    start -> Timer.Timer : [startTimer == true]
    (default) -> start
    Timer.Timer -> start [order 1] : [endTimer == true]
    Timer.TimeOut -> start
    Timer.Timer -> Timer.TimeOut [order 2] : [clock_Counter - t > (1300/prop)]
  state mainproc [parallel]
    settings: executionOrder=2
    state StandbyEquip
      entry:
      startTimer = true;
      endTimer = false;
    state MainEquip
    state TimeOut
    state wait4ACT
    note: 等待其他设备返回ACT
    note: 等待其他设备返回OK，receiver在接收到OK以后立马放弃主权
    state TempEquip
      entry:
      startTimer = true;
      endTimer = false;
    (default) -> StandbyEquip
    mainproc.TimeOut -> StandbyEquip
    StandbyEquip -> mainproc.TimeOut [order 2] : [timeOut == true]
    TempEquip -> StandbyEquip [order 1] : [BA == false]
        | {
        | endTimer = true;
        | startTimer = false;
        | }
    StandbyEquip -> MainEquip [order 1] : [BA == true && ACT == true]
        | {
        | endTimer = true;
        | startTimer = false;
        | }
    MainEquip -> wait4ACT : [acceptACT == true]
        | {
        | t = clock_Counter;
        | }
    TempEquip -> mainproc.TimeOut [order 2] : [timeOut == true]
    wait4ACT -> TempEquip : [acceptDomain == true]
        | {
        | t = clock_Counter;
        | }
  data: BA data_store_memory; ACT local boolean =true; acceptACT data_store_memory; acceptDomain data_store_memory; t local uint32; clock_Counter data_store_memory; startTimer local boolean; timeOut local boolean; endTimer local boolean; prop data_store_memory

== stateflow chart MVB1TestFlow/MVB2/Subsystem/Receiver ==
  state wait
  state wait4MFEnd
  note: acceptSF, acceptACT, acceptDomain在发送完主帧以后，根据主帧的类型进行相应的置位
      | 收到fcode为8的从帧之后，说明目标设备已经返回了OK，这时应该将ismaster设为1
  state judge4SF
  state judgeAddr
  note: 期待目标设备返回OK
  state wait4SF
  state wait4ACT
  state wait4Domain
  state MFReceive
  state MFcode0
  state MFcode8
  state MFcode15
  state STrans
  state MTrans
  (default) -> wait : {
      | t = clock_Counter;
      | }
  (junction 96) -> wait
  wait -> judge4SF [order 1] : [SFReceive== true]
      | {
      | t = 0;
      | }
  MTrans -> wait : [sendRandSFSign == false && sendOkSign == false && sendACTSign == false]
      | {
      | t = clock_Counter;
      | }
  wait -> wait4MFEnd [order 2] : [MFReceive==true]
  judgeAddr -> wait [order 2]
  wait4MFEnd -> judgeAddr : [MFReceive == false]
      | {fcodeIn = uint8(getFCode(MFIn));
      | addrIn = uint16(getAddr(MFIn));
      | t = 0;}
  judge4SF -> wait4Domain [order 3] : [acceptDomain == true]
  judge4SF -> (junction 96) [order 4]
  judge4SF -> wait4SF [order 1] : [acceptSF == true]
  STrans -> (junction 96) : [SFReceive == false]
  judge4SF -> wait4ACT [order 2] : [acceptACT == true]
  judgeAddr -> MFReceive [order 1] : [addrIn == LogicAddr]
  wait4SF -> STrans : {
      | acceptSF = false;
      | }
  wait4ACT -> STrans : [getbit(SFIn, 8)]
      | {
      | acceptACT = false;
      | }
  wait4Domain -> STrans : [getbit(SFIn, 16) == 1]
      | {
      | acceptDomain = false;
      | BA = false;
      | }
  MFReceive -> MFcode0 [order 2] : [fcodeIn == 0 && MFReceive == false ]
  MFReceive -> MFcode8 [order 3] : [fcodeIn == 8 && MFReceive == false]
  MFReceive -> MFcode15 [order 1] : [fcodeIn == 15 && MFReceive == false]
  MFcode0 -> MTrans : {sendRandSFSign = true}
  MFcode8 -> MTrans : {sendOkSign = true}
  MFcode15 -> MTrans : {sendACTSign = true}
  data: dataIn function_input uint32; num function_input uint32; r function_output uint32; dataIn function_input double; r function_output double; data function_input uint32; r function_output uint32; dataIn function_input double; r function_output double; r function_output uint32; data function_input uint32; MFIn input uint32; SFIn input uint32; t local uint32; clock_Counter data_store_memory; clock_3M data_store_memory; MFReceive input boolean; SFReceive input boolean; fcodeIn local uint8; addrIn local uint16; trans1 data_store_memory; LogicAddr data_store_memory; sendRandSFSign data_store_memory; sendOkSign data_store_memory; sendACTSign data_store_memory; acceptSF data_store_memory; acceptDomain data_store_memory; acceptACT data_store_memory; BA data_store_memory
  function r = getbit(dataIn, num):
    | function r = getbit(dataIn, num)
    | r = bitget(uint32(dataIn), num);
  function r = getFCode(dataIn):
    | function r = getFCode(dataIn)
    | % 右移12位 仅保留帧头和fcode
    | dataInExAddr = bitshift(uint32(dataIn), -12);
    | % 先右移16位再左移4位 仅仅保留帧头
    | dataInStart = bitshift(bitshift(uint32(dataIn), -16), 4);
    | % 相减得到fcode
    | r = double(dataInExAddr - dataInStart);
  function r = ManchesterEncoding(data):
    | function r = ManchesterEncoding(data)
    | r = data;
    | for i = 1:16
    |     x = bitget(data, i);
    |     if x == 0
    |         r = bitset(r, i*2-1, 1);
    |         r = bitset(r, i*2, 0);
    |     else
    |         r = bitset(r, i*2-1, 0);
    |         r = bitset(r, i*2, 1);
    |     end
    | end
  function r = getAddr(dataIn):
    | function r = getAddr(dataIn)
    | % 把后12位也就是地址归零
    | dataInExAddr = bitshift(bitshift(uint32(dataIn), -12), 12);
    | % 相减获取地址
    | r = double(dataIn - dataInExAddr);
  function r = ManchesterDecoding(data):
    | function r = ManchesterDecoding(data)
    | r = uint32(0);
    | for i = (1:2:32)
    |     x0 = bitget(data, i);
    |     x1 = bitget(data, i+1);
    |     if x0==0 && x1==1
    |         r = bitset(r, (i+1)/2, 1);
    |     else
    |         r = bitset(r, (i+1)/2, 0);
    |     end
    | end

== stateflow chart MVB1TestFlow/MVB3/Subsystem/Decoder ==
  state decodeSF
    decodeSF -> decodeSF [order 1] : CLK
        | {
        | ans = bitoperate.shiftbit(ans, 1) + SFIn;
        | count++;
        | }
  state bitoperate [group]
  state start
  state decodeMF
    decodeMF -> decodeMF [order 1] : CLK
        | {
        | ans = bitoperate.shiftbit(ans, 1) + MFIn;
        | count++;
        | }
  start -> decodeSF [order 2] : [SFInSign == true]
      | {
      | ans = 0;
      | count = 0;
      | SDataOut = 0;
      | SOutSign = true;
      | ans = bitoperate.shiftbit(ans, 1) + SFIn;
      | count++;
      | }
  decodeSF -> start [order 1] : [count==32]
      | {
      | ans = ManchesterDecoding(ans);
      | SDataOut = ans;
      | SOutSign = false;
      | }
  start -> decodeMF [order 1] : [MFInSign==true]
      | {
      | ans = 0;
      | count = 0;
      | MDataOut = 0;
      | MOutSign = true;
      | ans = bitoperate.shiftbit(ans, 1) + MFIn;
      | count++;
      | }
  (default) -> start
  decodeMF -> start [order 1] : [count==32]
      | {
      | ans = ManchesterDecoding(ans);
      | MDataOut = ans;
      | MOutSign = false;
      | }
  data: num function_input uint32; r function_output uint32; data function_input uint32; num function_input uint32; r function_output uint32; r function_output uint32; data function_input uint32; MFIn input uint32; SFIn input uint32; MDataOut output uint32; MFInSign input boolean; count local uint32; SFInSign input boolean; SDataOut output uint32; MOutSign output boolean; SOutSign output boolean; ans local uint32
  events: CLK input EITHER_EDGE_EVENT
  function r = getbit(num):
    | function r = getbit(num)
    | r = bitget(num, 32);
  function r = shiftbit(data, num):
    | function r = shiftbit(data, num)
    | r = bitshift(data, num);
    | %for i=1:cnt
    | %   r = bitset(r, i, 0);
    | %end
  function r = ManchesterDecoding(data):
    | function r = ManchesterDecoding(data)
    | r = uint32(0);
    | for i = (1:2:32)
    |     x0 = bitget(data, i);
    |     x1 = bitget(data, i+1);
    |     if x0==0 && x1==1
    |         r = bitset(r, (i+1)/2, 1);
    |     else
    |         r = bitset(r, (i+1)/2, 0);
    |     end
    | end

== stateflow chart MVB1TestFlow/MVB3/Subsystem/MainProc ==
  note: 上一个主帧接收后1.3ms没有收到主帧产生一个主帧超时的通知。
  state Timer [parallel]
    settings: executionOrder=1
    state Timer
      entry:
      t = clock_Counter;
      timeOut = false;
    state start
    state TimeOut
      entry:
      timeOut = true;
    start -> Timer.Timer : [startTimer == true]
    (default) -> start
    Timer.Timer -> start [order 1] : [endTimer == true]
    Timer.TimeOut -> start
    Timer.Timer -> Timer.TimeOut [order 2] : [clock_Counter - t > (1300/prop)]
  state mainproc [parallel]
    settings: executionOrder=2
    state StandbyEquip
      entry:
      startTimer = true;
      endTimer = false;
    state MainEquip
    state TimeOut
    state wait4ACT
    note: 等待其他设备返回ACT
    note: 等待其他设备返回OK，receiver在接收到OK以后立马放弃主权
    state TempEquip
      entry:
      startTimer = true;
      endTimer = false;
    (default) -> StandbyEquip
    mainproc.TimeOut -> StandbyEquip
    StandbyEquip -> mainproc.TimeOut [order 2] : [timeOut == true]
    TempEquip -> StandbyEquip [order 1] : [BA == false]
        | {
        | endTimer = true;
        | startTimer = false;
        | }
    StandbyEquip -> MainEquip [order 1] : [BA == true && ACT == true]
        | {
        | endTimer = true;
        | startTimer = false;
        | }
    MainEquip -> wait4ACT : [acceptACT == true]
        | {
        | t = clock_Counter;
        | }
    TempEquip -> mainproc.TimeOut [order 2] : [timeOut == true]
    wait4ACT -> TempEquip : [acceptDomain == true]
        | {
        | t = clock_Counter;
        | }
  data: BA data_store_memory; ACT local boolean =true; acceptACT data_store_memory; acceptDomain data_store_memory; t local uint32; clock_Counter data_store_memory; startTimer local boolean; timeOut local boolean; endTimer local boolean; prop data_store_memory

== stateflow chart MVB1TestFlow/MVB1/Subsystem/Receiver ==
  state wait
  state wait4MFEnd
  note: acceptSF, acceptACT, acceptDomain在发送完主帧以后，根据主帧的类型进行相应的置位
      | 收到fcode为8的从帧之后，说明目标设备已经返回了OK，这时应该将ismaster设为1
  state judge4SF
  state judgeAddr
  note: 期待目标设备返回OK
  state wait4SF
  state wait4ACT
  state wait4Domain
  state MFReceive
  state MFcode0
  state MFcode8
  state MFcode15
  state STrans
  state MTrans
  (default) -> wait : {
      | t = clock_Counter;
      | }
  (junction 96) -> wait
  wait -> judge4SF [order 1] : [SFReceive== true]
      | {
      | t = 0;
      | }
  MTrans -> wait : [sendRandSFSign == false && sendOkSign == false && sendACTSign == false]
      | {
      | t = clock_Counter;
      | }
  wait -> wait4MFEnd [order 2] : [MFReceive==true]
  judgeAddr -> wait [order 2]
  wait4MFEnd -> judgeAddr : [MFReceive == false]
      | {fcodeIn = uint8(getFCode(MFIn));
      | addrIn = uint16(getAddr(MFIn));
      | t = 0;}
  judge4SF -> wait4Domain [order 3] : [acceptDomain == true]
  judge4SF -> (junction 96) [order 4]
  judge4SF -> wait4SF [order 1] : [acceptSF == true]
  STrans -> (junction 96) : [SFReceive == false]
  judge4SF -> wait4ACT [order 2] : [acceptACT == true]
  judgeAddr -> MFReceive [order 1] : [addrIn == LogicAddr]
  wait4SF -> STrans : {
      | acceptSF = false;
      | }
  wait4ACT -> STrans : [getbit(SFIn, 8)]
      | {
      | acceptACT = false;
      | }
  wait4Domain -> STrans : [getbit(SFIn, 16) == 1]
      | {
      | acceptDomain = false;
      | BA = false;
      | }
  MFReceive -> MFcode0 [order 2] : [fcodeIn == 0 && MFReceive == false ]
  MFReceive -> MFcode8 [order 3] : [fcodeIn == 8 && MFReceive == false]
  MFReceive -> MFcode15 [order 1] : [fcodeIn == 15 && MFReceive == false]
  MFcode0 -> MTrans : {sendRandSFSign = true}
  MFcode8 -> MTrans : {sendOkSign = true}
  MFcode15 -> MTrans : {sendACTSign = true}
  data: dataIn function_input uint32; num function_input uint32; r function_output uint32; dataIn function_input double; r function_output double; data function_input uint32; r function_output uint32; dataIn function_input double; r function_output double; r function_output uint32; data function_input uint32; MFIn input uint32; SFIn input uint32; t local uint32; clock_Counter data_store_memory; clock_3M data_store_memory; MFReceive input boolean; SFReceive input boolean; fcodeIn local uint8; addrIn local uint16; trans1 data_store_memory; LogicAddr data_store_memory; sendRandSFSign data_store_memory; sendOkSign data_store_memory; sendACTSign data_store_memory; acceptSF data_store_memory; acceptDomain data_store_memory; acceptACT data_store_memory; BA data_store_memory
  function r = getbit(dataIn, num):
    | function r = getbit(dataIn, num)
    | r = bitget(uint32(dataIn), num);
  function r = getFCode(dataIn):
    | function r = getFCode(dataIn)
    | % 右移12位 仅保留帧头和fcode
    | dataInExAddr = bitshift(uint32(dataIn), -12);
    | % 先右移16位再左移4位 仅仅保留帧头
    | dataInStart = bitshift(bitshift(uint32(dataIn), -16), 4);
    | % 相减得到fcode
    | r = double(dataInExAddr - dataInStart);
  function r = ManchesterEncoding(data):
    | function r = ManchesterEncoding(data)
    | r = data;
    | for i = 1:16
    |     x = bitget(data, i);
    |     if x == 0
    |         r = bitset(r, i*2-1, 1);
    |         r = bitset(r, i*2, 0);
    |     else
    |         r = bitset(r, i*2-1, 0);
    |         r = bitset(r, i*2, 1);
    |     end
    | end
  function r = getAddr(dataIn):
    | function r = getAddr(dataIn)
    | % 把后12位也就是地址归零
    | dataInExAddr = bitshift(bitshift(uint32(dataIn), -12), 12);
    | % 相减获取地址
    | r = double(dataIn - dataInExAddr);
  function r = ManchesterDecoding(data):
    | function r = ManchesterDecoding(data)
    | r = uint32(0);
    | for i = (1:2:32)
    |     x0 = bitget(data, i);
    |     x1 = bitget(data, i+1);
    |     if x0==0 && x1==1
    |         r = bitset(r, (i+1)/2, 1);
    |     else
    |         r = bitset(r, (i+1)/2, 0);
    |     end
    | end
